simulink model "lqr_lin"  (R2024b)
settings: Solver=VariableStepAuto  StartTime=0.0  StopTime=params.simtime  RelTol=1e-3
values from neighbouring files (symbols this model uses):
  params = parameters()    [lqr_compare.m]    (also in lqr_pil.m)
undefined symbols (not defined in the file or in its folder): lin_model
settings Model: Creator=ben83  LastModifiedBy=ben
settings RTWCC: GPUComputeCapability=3.5

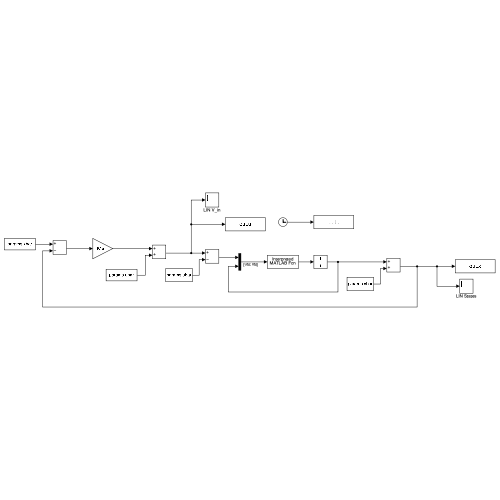
[thumbnail: Simulink's stored preview of the top-level diagram]
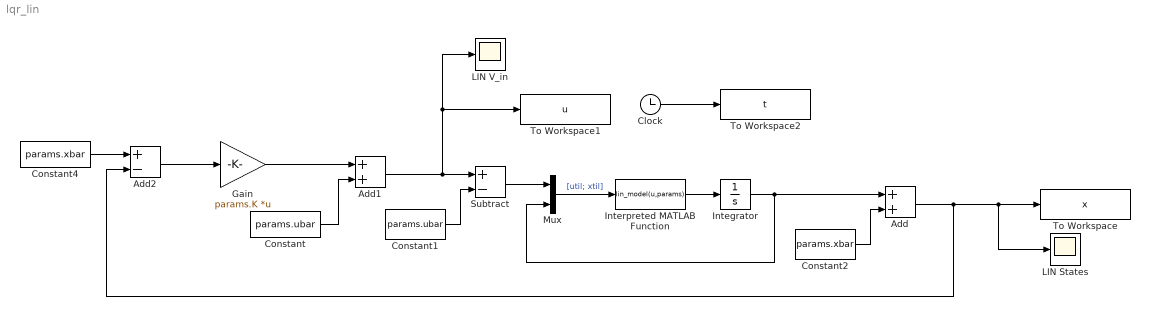
== system lqr_lin ==
  Add : Sum
  Add1 : Sum
  Add2 : Sum  Inputs=+-
  Clock : Clock
  Constant : Constant  Value=params.ubar
  Constant1 : Constant  Value=params.ubar
  Constant2 : Constant  Value=params.xbar
  Constant4 : Constant  Value=params.xbar
  Gain : Gain  Gain=params.K  Multiplication=Matrix(K*u)
  Integrator : Integrator  InitialCondition=params.iclin
  Interpreted MATLAB Function : MATLABFcn  MATLABFcn=lin_model(u,params)
  LIN States : Scope
  LIN V_in : Scope
  Mux : Mux  Inputs=2
  Subtract : Sum  Inputs=+-
  To Workspace : ToWorkspace  VariableName=x  SampleTime=-1
  To Workspace1 : ToWorkspace  VariableName=u  SampleTime=-1
  To Workspace2 : ToWorkspace  VariableName=t  SampleTime=-1
  wires:
  Interpreted MATLAB Function/1 -> Integrator/1
  Mux/1 -> Interpreted MATLAB Function/1  "[util; xtil]"
  Clock/1 -> To Workspace2/1
  Integrator/1 -> Add/1, Mux/2
  Subtract/1 -> Mux/1
  Add1/1 -> LIN V_in/1, To Workspace1/1, Subtract/1
  Constant1/1 -> Subtract/2
  Constant2/1 -> Add/2
  Gain/1 -> Add1/1
  Constant/1 -> Add1/2
  Add/1 -> Add2/2, LIN States/1, To Workspace/1
  Constant4/1 -> Add2/1
  Add2/1 -> Gain/1
